simulink model "pendulum_model"  (R2025b)
settings: Solver=VariableStepAuto  StartTime=0.0  StopTime=20  RelTol=1e-3
undefined symbols (not defined in the file): b, K, L, R
settings Model: Creator=REARDONNM24  LastModifiedBy=REARDONNM24

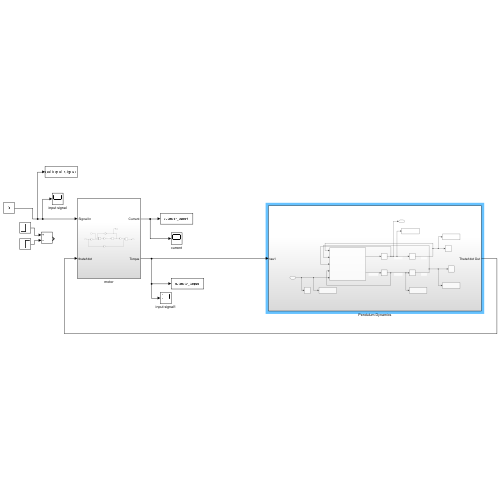
[thumbnail: Simulink's stored preview of the top-level diagram]
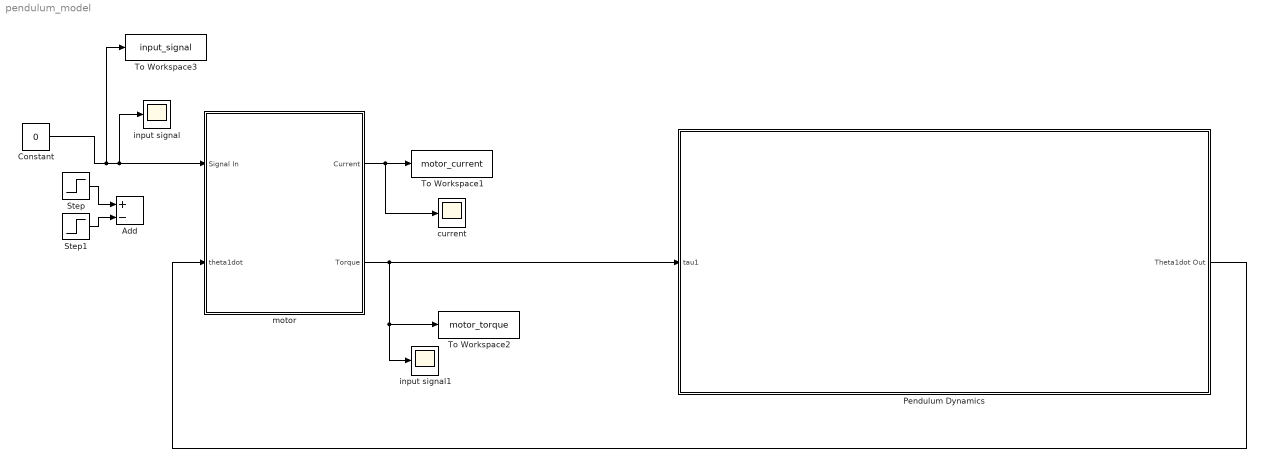
== system pendulum_model ==
  Add : Sum  Inputs=+-
  Constant : Constant  Value=0
  Pendulum Dynamics : Subsystem
  Step : Step  After=10  SampleTime=0
  Step1 : Step  Time=2  After=10  SampleTime=0
  To Workspace1 : ToWorkspace  VariableName=motor_current  SaveFormat=Timeseries  SampleTime=-1
  To Workspace2 : ToWorkspace  VariableName=motor_torque  SaveFormat=Timeseries  SampleTime=-1
  To Workspace3 : ToWorkspace  VariableName=input_signal  SaveFormat=Timeseries  SampleTime=-1
  current : Scope
      settings: ActiveDisplayYMinimum=174.41543511722466  ActiveDisplayYMaximum=4357.1108128089754  DataLoggingVariableName=ScopeData5
  input signal : Scope
      settings: ActiveDisplayYMinimum=174.41543511722466  ActiveDisplayYMaximum=4357.1108128089754  DataLoggingVariableName=ScopeData6
  input signal1 : Scope
      settings: ActiveDisplayYMinimum=-0.0033441907118329393  ActiveDisplayYMaximum=0.00610606731194419  DataLoggingVariableName=ScopeData7
  motor : Subsystem
  wires:
  motor/1(Current) -> current/1, To Workspace1/1
  motor/2(Torque) -> To Workspace2/1, input signal1/1, Pendulum Dynamics/1(tau1)
  Pendulum Dynamics/1(Theta1dot Out) -> motor/2(theta1dot)
  Step/1 -> Add/1
  Step1/1 -> Add/2
  Constant/1 -> To Workspace3/1, input signal/1, motor/1(Signal In)

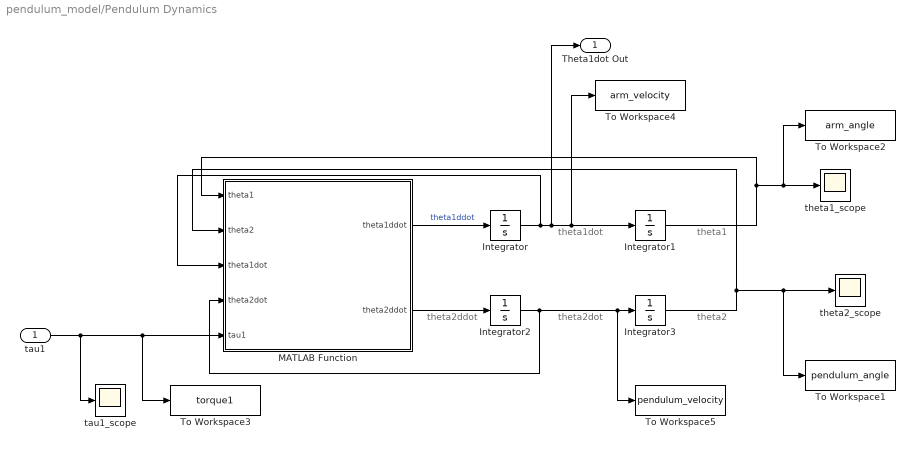
== system pendulum_model/Pendulum Dynamics ==
  note: theta1
  note: theta2
  note: theta2dot
  note: theta2ddot
  note: theta1dot
  tau1 : Inport
  Integrator : Integrator
  Integrator1 : Integrator
  Integrator2 : Integrator
  Integrator3 : Integrator  InitialCondition=2
  MATLAB Function : MATLAB Function  TreatAsAtomicUnit=on
  To Workspace1 : ToWorkspace  VariableName=pendulum_angle  SaveFormat=Timeseries  SampleTime=-1
  To Workspace2 : ToWorkspace  VariableName=arm_angle  SaveFormat=Timeseries  SampleTime=-1
  To Workspace3 : ToWorkspace  VariableName=torque1  SaveFormat=Timeseries  SampleTime=-1
  To Workspace4 : ToWorkspace  VariableName=arm_velocity  SaveFormat=Timeseries  SampleTime=-1
  To Workspace5 : ToWorkspace  VariableName=pendulum_velocity  SaveFormat=Timeseries  SampleTime=-1
  tau1_scope : Scope
      settings: ActiveDisplayYMinimum=-0.018770395001535239  ActiveDisplayYMaximum=0.012159767110327464  DataLoggingVariableName=ScopeData4
  theta1_scope : Scope
      settings: ActiveDisplayYMinimum=-0.0042282998397400089  ActiveDisplayYMaximum=0.03805469855766009  DataLoggingVariableName=ScopeData2
  theta2_scope : Scope
      settings: ActiveDisplayYMinimum=-1.85410777692418  ActiveDisplayYMaximum=-0.63109346273532874  DataLoggingVariableName=ScopeData3
  Theta1dot Out : Outport
  wires:
  MATLAB Function/1(theta1ddot) -> Integrator/1  "theta1ddot"
  Integrator/1 -> MATLAB Function/3(theta1dot), Theta1dot Out/1, Integrator1/1, To Workspace4/1
  Integrator2/1 -> MATLAB Function/4(theta2dot), To Workspace5/1, Integrator3/1
  MATLAB Function/2(theta2ddot) -> Integrator2/1
  Integrator3/1 -> To Workspace1/1, theta2_scope/1, MATLAB Function/2(theta2)
  Integrator1/1 -> To Workspace2/1, theta1_scope/1, MATLAB Function/1(theta1)
  tau1/1 -> tau1_scope/1, To Workspace3/1, MATLAB Function/5(tau1)

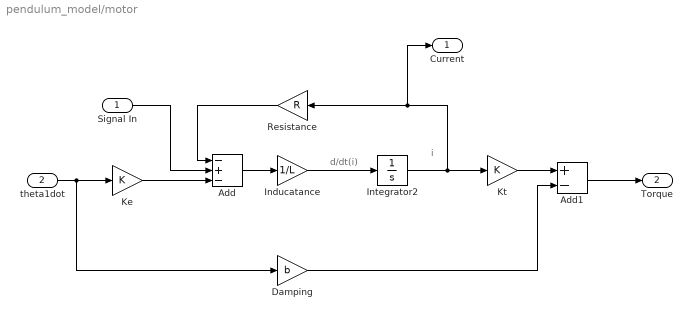
== system pendulum_model/motor ==
  note: i
  note: d/dt(i)
  Signal In : Inport
  theta1dot : Inport  Port=2
  Add : Sum  Inputs=-+-
  Add1 : Sum  Inputs=+-
  Damping : Gain  Gain=b
  Inducatance : Gain  Gain=1/L
  Integrator2 : Integrator
  Ke : Gain  Gain=K
  Kt : Gain  Gain=K
  Resistance : Gain  Gain=R
  Current : Outport
  Torque : Outport  Port=2
  wires:
  Signal In/1 -> Add/2
  Resistance/1 -> Add/1
  Integrator2/1 -> Kt/1, Current/1, Resistance/1
  Inducatance/1 -> Integrator2/1
  Add/1 -> Inducatance/1
  Ke/1 -> Add/3
  theta1dot/1 -> Damping/1, Ke/1
  Kt/1 -> Add1/1
  Damping/1 -> Add1/2
  Add1/1 -> Torque/1

== matlab function pendulum_model/Pendulum Dynamics/MATLAB Function ==
  data: theta1 input; theta1ddot output; theta2 input; theta1dot input; theta2dot input; tau1 input; theta2ddot output
function [theta1ddot, theta2ddot] = pendulum_dynamics(theta1, theta2, theta1dot, theta2dot, tau1)
    % Define constants
    L1 = 0.278;
    % L2 = 0.3;
    L2 = 0.05;
    l1 = 0.15;
    l2 = 0.148;
    m1 = 0.3;
    m2 = 0.075;
    J1 = 2.48e-2;
    J2 = 3.86e-3;
    b1 = 1e-4;
    b2 = 2.8e-4;
    g = 9.81;

    % assume the following for now:
    J1xx = 0;
    J1yy = J1;
    J1zz = J1;
    J2xx = 0;
    J2yy = J2;
    J2zz = J2;

    % define the mass matrix
    M11 = J1zz + m1*l1^2 + m2*L1^2 + (J2yy+m2*l2^2)*sin(theta2)^2 + J2xx*cos(theta2)^2;
    M12 = m2*L1*l2*cos(theta2);
    M22 = m2*l2^2 + J2zz;

    M = [M11, M12; M12, M22];
    
    h1 = -m2*L1*l2*sin(theta2)*theta2dot^2 + theta1dot*theta2dot*sin(2*theta2)*(m2*l2^2 + J2yy - J2xx) + b1*theta1dot;
    h2 = 0.5*theta1dot^2*sin(2*theta2)*(-m2*l2^2 - J2yy + J2xx) + b2*theta2dot + g*m2*l2*sin(theta2);
    

    tau = [tau1; 0];

        
    qdd = M\(tau - [h1;h2]);

    theta1ddot = qdd(1);
    theta2ddot = qdd(2);
  

end
